simulink model "DC-Motor-Control"  (R2024a)
settings: Solver=VariableStepAuto  StartTime=0.0  StopTime=10  MaxStep=1e-5  RelTol=1e-7  AbsTol=1e-7
values from neighbouring files (symbols this model uses):
  J = 5    [Parameters.m]    (also in project1.m)
  Ke = 3.65    [Parameters.m]    (also in project1.m)
  kii = (2*pi*fsw*Ra)/(10*Vg)    (= 0.0816814089933)    [Parameters.m]    (also in project1.m)
  kiw = kpw/((a*a)*(te+tauf))    [Parameters.m]    (also in project1.m)
  kpi = (2*pi*fsw*La)/(10*Vg)    (= 0.00157079632679)    [Parameters.m]    (also in project1.m)
  kpw = J/(a*Ke*(te+tauf))    [Parameters.m]    (also in project1.m)
  La = 1e-3    (= 0.001)    [Parameters.m]    (also in project1.m)
  Ra = 0.052    [Parameters.m]    (also in project1.m)
  tauf = 1/(2*pi*10)    (= 0.0159154943092)    [Parameters.m]    (also in project1.m)
  Vg = 800    [Parameters.m]    (also in project1.m)
  wmr = 1250    [Parameters.m]    (also in project1.m)
libraries: spsIGBTDiodeLib x4, spsCurrentMeasurementLib x1, spsDCMachineLib x1, spsDCVoltageSourceLib x1, simulink x1, sps_lib x1
settings Model: Creator=akash  LastModifiedBy=Rhythm Shah

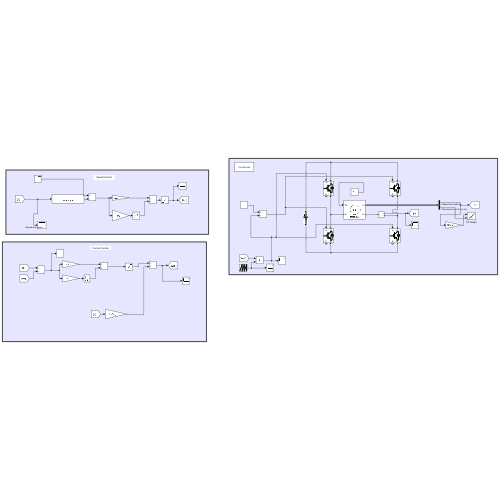
[thumbnail: Simulink's stored preview of the top-level diagram]
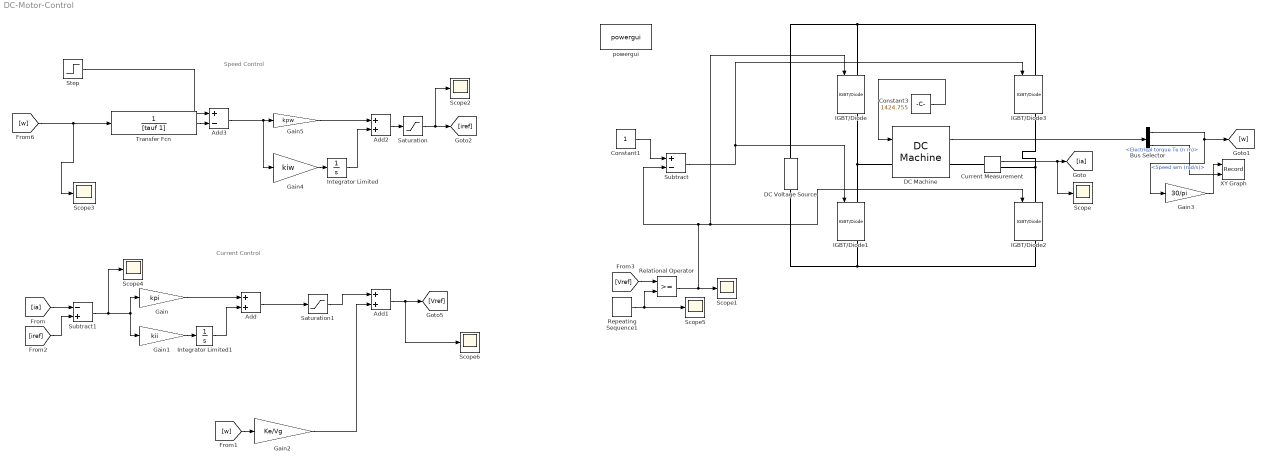
== system DC-Motor-Control ==
  note: Speed Control
  note: Current Control
  Add : Sum
  Add1 : Sum
  Add2 : Sum
  Add3 : Sum  Inputs=+-
  Bus Selector : BusSelector  OutputSignals=Speed wm (rad/s),Electrical torque Te (n m)
  Constant1 : Constant
  Constant3 : Constant  Value=1424.755
  Current Measurement : spsCurrentMeasurementLib/Current Measurement  PhasorSimulation=off  OutputType=Complex  PSBequivalent=0
  DC Machine : spsDCMachineLib/DC Machine  PresetModel=No  MechanicalLoad=Torque TL  FieldType=Permanent magnet  ShowDetailedParameters=on  MeasurementBus=off  RLa="[ Ra  La]"  RLf="[ 240  120]"  Laf=1.8  MachineConstant=Torque constant (N.m/A)  Ke=1.8  Kt=Ke  J=J  Bm=0  Tf=0  w0=0  Ifinit=1  TsPowergui=0  TsBlock=-1
  DC Voltage Source : spsDCVoltageSourceLib/DC Voltage Source  Amplitude=800  Measurements=None
  Gain : Gain  Gain=kpi
  Gain1 : Gain  Gain=kii
  Gain2 : Gain  Gain=Ke/Vg
  Gain3 : Gain  Gain=30/pi
  Gain4 : Gain  Gain=kiw
  Gain5 : Gain  Gain=kpw
  IGBT/Diode{,1..3} (4 alike) : spsIGBTDiodeLib/IGBT//Diode  Ron=0  Rs=inf  Cs=inf  Measurements=on
  Integrator Limited : Integrator  LimitOutput=on  UpperSaturationLimit=500  LowerSaturationLimit=-500
  Integrator Limited1 : Integrator  LimitOutput=on  UpperSaturationLimit=1  LowerSaturationLimit=-1
  Relational Operator : RelationalOperator  OutDataTypeStr=boolean  RndMeth=Simplest  InputSameDT=off
  Repeating Sequence1 : simulink/Sources/Repeating Sequence  rep_seq_t=[0 0.0005]  rep_seq_y=[-1 1]
  Saturation : Saturate  UpperLimit=500  LowerLimit=-500
  Saturation1 : Saturate  UpperLimit=1  LowerLimit=-1
  Scope{,1..6} (7 alike) : Scope
  Step : Step  Time=0  After=wmr  SampleTime=0
  Subtract : Sum  Inputs=+-
  Subtract1 : Sum  Inputs=-+
  Transfer Fcn : TransferFcn  Denominator=[tauf 1]
  XY Graph : Record  FileSettingsInternal="{\"entries\":[{\"content\":{\"excelSettings\":{\"content\":{},\"type\":\"Streamout.ExcelSettings\"}},\"type\":\"Streamout.FileSettingStorage\",\"uuid\":\"\"}],\"packageUris\":[\"http:\\/\\/schema.mathworks.com\\/mf0\\/streamout_blocks\\/R2020a\"],\"version\":\"1.0\"}"  Layout=[1 1]  SignalsInternal="{\"entries\":[{\"content\":{\"signals\":[{\"content\":{\"blockPath\":[],\"dimensions\":[1],\"domain\":\"\",\"lineColor\":\"#a2142f\",\"plots\":[ 1 ],\"port\":1,\"sid\":[\"\"],\"signalID\":1,\"signalName\":\"Gain3\"},\"type\":\"RecordBlkView.Signal\",\"uuid\":\"\"},{\"content\":{\"blockPath\":[],\"dimensions\":[1],\"domain\":\"\",\"lineColor\":\"#139fff\",\"plots\":[ 1 ],\"port\":2,\"sid\":[\"\"],\"signalID\":2,\"signalName\":\"<Electrical torque Te (n m)>\"},\"type\":\"RecordBlkView.Signal\",\"uuid\":\"\"}]},\"type\":\"RecordBlkView.InputSignals\",\"uuid\":\"\"}],\"packageUris\":[\"http:\\/\\/schema.mathworks.com\\/mf0\\/streamout_blocks\\/R2020a\"],\"version\":\"1.0\"}"  VisualizationBindings="{\"xyplotplugin\":{\"info\":[{\"series\":[{\"bindingParametersList\":[{\"parameter\":\"X-Axis\",\"signalID\":1,\"signalName\":\"Gain3\"},{\"parameter\":\"Y-Axis\",\"signalID\":2,\"signalName\":\"<Electrical torque Te (n m)>\"}],\"seriesID\":0}],\"subplotID\":1}]}}"  CompatibilityTag=XY
  powergui : sps_lib/powergui  Priority=1  SimulationMode=Continuous  SampleTime=10e-3  frequency=60  Iterations=50  frequencyindice=0  Pbase=100e6  ErrMax=1e-4  UnitsV=kV  UnitsW=MW  buscounter=0  FunctionMessages=off  echomessages=off  EnableUseOfTLC=off  CurrentSourceSwitches=off  DisableSnubberDevices=off  DisableRonSwitches=off  DisableVfSwitches=off  DisplayEquations=off  AutomaticDiscreteSolvers=off  SolverType=Tustin/Backward Euler (TBE)  Interpol=off  ExternalGateDelay=off  methode=off  Ts=100  x0status=blocks  SPID=on  SwTol=0  HookPort=off  NonlinearTolerance=1e-4  nMaxIteration=100  ContinueOnMaxIteration=off  RestoreLinks=warning  ResistiveCurrentMeasurement=off  Frange=[0:2:500]  Ylog=off  Xlog=on  ShowGrid=off  save=off  variable=ZData  structure=0  ZoomFFT=off  StartTime=0.0  cycles=1  DisplayStyle=1  fundamental=60  FreqAxis=off  MaxFrequency=1000  frequencyindicesteady=1  RmsSteady=1  display=off
  wires:
  Relational Operator/1 -> Subtract/2, IGBT/Diode2/1, IGBT/Diode/1, Scope1/1
  Constant1/1 -> Subtract/1
  Subtract/1 -> IGBT/Diode1/1, IGBT/Diode3/1
  DC Machine/1 -> Bus Selector/1
  Bus Selector/1 -> Gain3/1, [w]  "<Speed wm (rad/s)>"
  Repeating Sequence1/1 -> Scope5/1, Relational Operator/2
  Constant3/1 -> DC Machine/1
  Current Measurement/1 -> Scope/1, [ia]
  [Vref] -> Relational Operator/1
  [w] -> Gain2/1
  [iref] -> Subtract1/2
  Add/1 -> Saturation1/1
  Gain/1 -> Add/1
  Gain2/1 -> Add1/2
  Saturation1/1 -> Add1/1
  [ia] -> Subtract1/1
  Add1/1 -> [Vref], Scope6/1
  Integrator Limited1/1 -> Add/2
  Gain1/1 -> Integrator Limited1/1
  Transfer Fcn/1 -> Add3/2
  Gain5/1 -> Add2/1
  Add3/1 -> Gain4/1, Gain5/1
  Step/1 -> Add3/1
  Add2/1 -> Saturation/1
  Gain4/1 -> Integrator Limited/1
  Integrator Limited/1 -> Add2/2
  Saturation/1 -> Scope2/1, [iref]
  [w] -> Transfer Fcn/1, Scope3/1
  Subtract1/1 -> Scope4/1, Gain1/1, Gain/1
  Bus Selector/2 -> XY Graph/2  "<Electrical torque Te (n m)>"
  Gain3/1 -> XY Graph/1
  connections:
  DC Voltage Source/RConn1 -- IGBT/Diode3/LConn1 -- IGBT/Diode/LConn1
  IGBT/Diode/RConn1 -- DC Machine/LConn1 -- IGBT/Diode1/LConn1
  IGBT/Diode1/RConn1 -- DC Voltage Source/LConn1 -- IGBT/Diode2/RConn1
  DC Machine/RConn1 -- Current Measurement/LConn1
  IGBT/Diode2/LConn1 -- Current Measurement/RConn1 -- IGBT/Diode3/RConn1
